simulink model "Copy_of_Robot_PID_Trajectory_Control"  (R2019b)
settings: Solver=VariableStepAuto  StartTime=0.0  StopTime=6  RelTol=1e-3  EnableMultiTasking=on
model workspace: external: MATLAB File D:\Google Drive\Duongw_Folder\Thesis Master\_Model\Delta_Model_ADEPT\SIMCAPE_MULTI_BODY\ADEPT_DELTA_3AXES1\Assem1_ADEPT_HORNET_DataFile.m (data not in the file)
values from neighbouring files (symbols this model uses):
  G = -5    [Assem1_ADEPT_HORNET_DataFile.m]    (also in data_specMotor.m)
  Kb = 0.4    [Assem1_ADEPT_HORNET_DataFile.m]    (also in data_specMotor.m)
  Kd = 15    [Assem1_ADEPT_HORNET_DataFile.m]    (also in data_specMotor.m)
  Ki = 200    [Assem1_ADEPT_HORNET_DataFile.m]    (also in data_specMotor.m)
  Km = 0.7    [Assem1_ADEPT_HORNET_DataFile.m]    (also in data_specMotor.m)
  Kp = 300    [Assem1_ADEPT_HORNET_DataFile.m]    (also in data_specMotor.m)
  La = 0.0062000000000000006    (= 0.0062)    [Assem1_ADEPT_HORNET_DataFile.m]    (also in data_specMotor.m)
  m = zeros(1,3)    [forward.m]    (also in solequa.m = zeros(3,1))
  Ra = 1.8    [Assem1_ADEPT_HORNET_DataFile.m]    (also in data_specMotor.m)
  smiData = struct    [Assem1_ADEPT_HORNET_DataFile.m]
undefined symbols (not defined in the file or in its folder): X, Y, Z
libraries: sm_lib x106, nesl_utility x7
(part 1 of 4)
settings Model: Creator=ThanhUTC  LastModifiedBy=ShiningDanyang
settings DataIOCC: SaveFormat=Array  ReturnWorkspaceOutputs=off
settings OptimizationCC: LifeSpan=inf
settings DebuggingCC: SFUnexpectedBacktrackingDiag=warning  SFNoUnconditionalDefaultTransitionDiag=warning  SFExecutionAtInitializationDiag=none  ArithmeticOperatorsInVariantConditions=warning
settings SFSimCC: SimUseLocalCustomCode=off  CustomCodeUndefinedFunction=UseInterfaceOnly
settings RTWCC: RTWUseLocalCustomCode=off
settings CodeAppCC: StateflowObjectComments=on
settings GRTTargetCC: TargetLangStandard=C89/C90 (ANSI)
settings ConfigComp: CovMetricSettings=dw  CovHtmlReporting=on  CovSaveCumulativeToWorkspaceVar=on  CovSaveSingleToWorkspaceVar=on  CovExternalEMLEnable=off
settings SimscapeCC: SimscapeNormalizeSystem=off
settings ExplorerConfigSet: InternalSimMechanicsExplorerSettings="<ExplorerConfiguration><canonicalview>aerospace</canonicalview><AnimationSetting><BasePlaybackSpeed>1.0</BasePlaybackSpeed><PlaybackSpeedFactor>1.0</PlaybackSpeedFactor></AnimationSetting><TilePanel><TileInfo><Tiles Columns=\"2\" Count=\"4\" Rows=\"2\"><Column Left=\"2\" Weight=\"0.5\"/><Column Left=\"475\" Weight=\"0.5\"/><Column Left=\"948\"/><Row Top=\"2\" Weight=\"0.4991\"/><Row Top=\"300\" Weight=\"0.5009\"/><Row Top=\"599\"/><Tile Height=\"1\" Width=\"1\" X=\"0\" Y=\"0\"/><Tile Height=\"1\" Width=\"1\" X=\"0\" Y=\"1\"/><Tile Height=\"1\" Width=\"1\" X=\"1\" Y=\"0\"/><Tile Height=\"1\" Width=\"1\" X=\"1\" Y=\"1\"/></Tiles></TileInfo><SceneInfo><SceneViewer><BGColor><R>0.60000002384185791</R><G>0.60000002384185791</G><B>0.60000002384185791</B></BGColor><Camera><DoPerspective>off</DoPerspective><Position><X>0.70243808377411976</X><Y>0.13073659989605124</Y><Z>0.39252081211592249</Z></Position><Center><X>-0.2309184998542182</X><Y>0.13073659989605124</Y><Z>0.39252081211592249</Z></Center><Up><X>0</X><Y>0</Y><Z>-1</Z></Up><ViewLimDist>1</ViewLimDist><YLim>0.65085916161537172</YLim><XLim>1.0449780311056487</XLim></Camera></SceneViewer><SceneViewer><BGColor><R>0.60000002384185791</R><G>0.60000002384185791</G><B>0.60000002384185791</B></BGColor><Camera><DoPerspective>off</DoPerspective><Position><X>-0.23091849925817176</X><Y>0.13073659989605124</Y><Z>-0.77434821586150304</Z></Position><Center><X>-0.23091849925817176</X><Y>0.13073659989605124</Y><Z>0.3925208407261519</Z></Center><Up><X>0</X><Y>-1</Y><Z>0</Z></Up><ViewLimDist>1</ViewLimDist><YLim>0.42854619026184082</YLim><XLim>0.68567390441894538</XLim></Camera></SceneViewer><SceneViewer><BGColor><R>0.60000002384185791</R><G>0.60000002384185791</G><B>0.60000002384185791</B></BGColor><Camera><DoPerspective>off</DoPerspective><Position><X>-0.23091849925817176</X><Y>-0.77390347671190962</Y><Z>0.39252081211592216</Z></Position><Center><X>-0.23091849925817176</X><Y>0.13073658559093626</Y><Z>0.39252081211592216</Z></Center><Up><X>0</X><Y>0</Y><Z>-1</Z></Up><ViewLimDist>1</ViewLimDist><YLim>0.65085916161537172</YLim><XLim>1.0449780311056487</XLim></Camera></SceneViewer><SceneViewer><BGColor><R>0.60000002384185791</R><G>0.60000002384185791</G><B>0.60000002384185791</B></BGColor><Camera><DoPerspective>off</DoPerspective><Position><X>0.27338855069047568</X><Y>-0.44960389100580933</Y><Z>-0.34981142573849433</Z></Position><Center><X>-0.23784198094965553</X><Y>0.061626640634321911</Y><Z>0.16141910590163688</Z></Center><Up><X>-0.40824829046386307</X><Y>0.40824829046386307</Y><Z>-0.81649658092772615</Z></Up><ViewLimDist>1</ViewLimDist><YLim>0.7367131638526917</YLim><XLim>1.1787410621643069</XLim></Camera></SceneViewer></SceneInfo></TilePanel><MechEditorPanel><Cameras/><GfxPanelCameraMap/></MechEditorPanel></ExplorerConfiguration>"

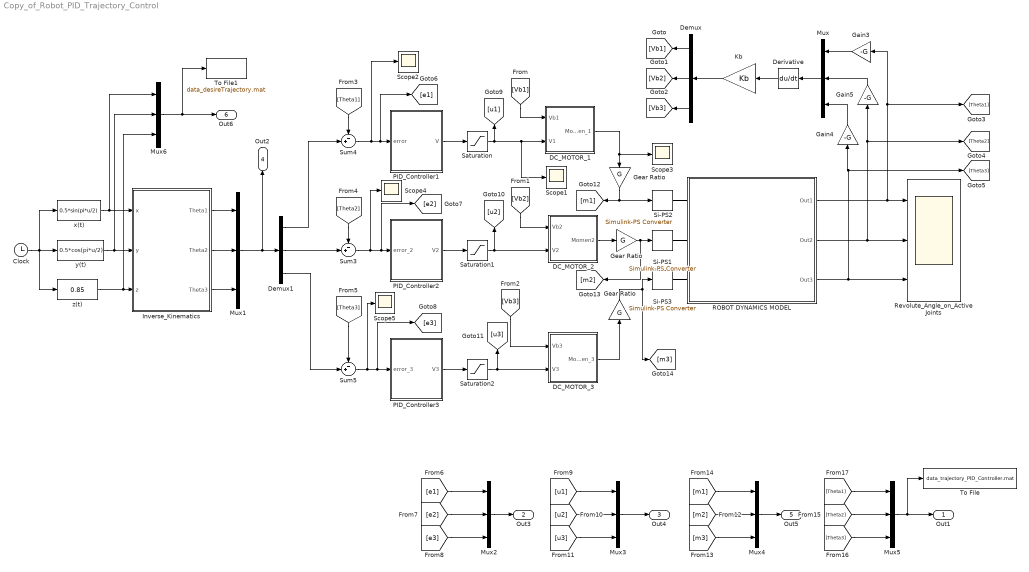
== system Copy_of_Robot_PID_Trajectory_Control ==
  Clock : Clock
  DC_MOTOR_1 : Subsystem
  DC_MOTOR_2 : Subsystem
  DC_MOTOR_3 : Subsystem
  Demux : Demux  Outputs=3
  Demux1 : Demux  Outputs=3
  Derivative : Derivative
  Gain3 : Gain  Gain=-G
  Gain4 : Gain  Gain=-G
  Gain5 : Gain  Gain=-G
  Gear Ratio : Gain  Gain=G
  Gear Ratio : Gain  Gain=G
  "Gear Ratio " : Gain  Gain=G
  Inverse_Kinematics : Subsystem
  Kb : Gain  Gain=Kb
  Mux{,1..6} (7 alike) : Mux  Inputs=3
  PID_Controller1 : Subsystem
  PID_Controller2 : Subsystem
  PID_Controller3 : Subsystem
  ROBOT DYNAMICS MODEL : Subsystem
  Revolute_Angle_on_Active Joints : Scope  NumInputPorts=3
  Saturation : Saturate  UpperLimit=40  LowerLimit=-40  ZeroCross=off
  Saturation1 : Saturate  UpperLimit=40  LowerLimit=-40  ZeroCross=off
  Saturation2 : Saturate  UpperLimit=40  LowerLimit=-40  ZeroCross=off
  Scope{1..5} (5 alike) : Scope
  Si-PS1 : nesl_utility/Simulink-PS Converter  PhysicalDomain=network_engine_domain  SubClassName=ps_input  LeftPortType=input  RightPortType=output  PseudoPeriodic=off  Frequencies=[]  NoiseDistribution=none  NoiseParameters=[]  Unit=1  AffineConversion=off  FilteringAndDerivatives=filter  SimscapeFilterOrder=2  InputFilterTimeConstant=0.001  UdotUserProvided=1
  Si-PS2 : nesl_utility/Simulink-PS Converter  PhysicalDomain=network_engine_domain  SubClassName=ps_input  LeftPortType=input  RightPortType=output  PseudoPeriodic=off  Frequencies=[]  NoiseDistribution=none  NoiseParameters=[]  Unit=1  AffineConversion=off  FilteringAndDerivatives=filter  SimscapeFilterOrder=2  InputFilterTimeConstant=0.001  UdotUserProvided=1
  Si-PS3 : nesl_utility/Simulink-PS Converter  PhysicalDomain=network_engine_domain  SubClassName=ps_input  LeftPortType=input  RightPortType=output  PseudoPeriodic=off  Frequencies=[]  NoiseDistribution=none  NoiseParameters=[]  Unit=1  AffineConversion=off  FilteringAndDerivatives=filter  SimscapeFilterOrder=2  InputFilterTimeConstant=0.001  UdotUserProvided=1
  Sum3 : Sum  Inputs=-+|
  Sum4 : Sum  Inputs=-+|
  Sum5 : Sum  Inputs=-+|
  To File : ToFile  Filename=data_trajectory_PID_Controller.mat
  To File1 : ToFile  Filename=data_desireTrajectory.mat  MatrixName=xyz_d
  x(t) : Fcn  Expr=0.5*sin(pi*u/2)
  y(t) : Fcn  Expr=0.5*cos(pi*u/2)
  z(t) : Fcn  Expr=0.85
  Out1 : Outport  VectorParamsAs1DForOutWhenUnconnected=off
  Out3 : Outport  Port=2  VectorParamsAs1DForOutWhenUnconnected=off
  Out4 : Outport  Port=3  VectorParamsAs1DForOutWhenUnconnected=off
  Out2 : Outport  Port=4  VectorParamsAs1DForOutWhenUnconnected=off
  Out5 : Outport  Port=5  VectorParamsAs1DForOutWhenUnconnected=off
  Out6 : Outport  Port=6  VectorParamsAs1DForOutWhenUnconnected=off
  wires:
  Mux/1 -> Derivative/1
  Derivative/1 -> Kb/1
  Kb/1 -> Demux/1
  Demux/1 -> [Vb1]
  Demux/2 -> [Vb2]
  Demux/3 -> [Vb3]
  [Theta1] -> Sum4/1
  [Vb1] -> DC_MOTOR_1/1(Vb1)
  PID_Controller1/1("V ") -> Saturation/1
  DC_MOTOR_1/1(Momen_1) -> Scope3/1, Gear Ratio/1
  [Theta2] -> Sum3/1
  Sum3/1 -> Scope4/1, [e2], PID_Controller2/1(error_2)
  PID_Controller2/1("V2 ") -> Saturation1/1
  [Theta3] -> Sum5/1
  Sum5/1 -> Scope5/1, [e3], PID_Controller3/1(error_3)
  PID_Controller3/1("V3 ") -> Saturation2/1
  [Vb2] -> DC_MOTOR_2/1(Vb2)
  DC_MOTOR_2/1(Momen2) -> Gear Ratio/1
  [Vb3] -> DC_MOTOR_3/1(Vb3)
  DC_MOTOR_3/1(Momen_3) -> "Gear Ratio "/1
  "Gear Ratio "/1 -> [m3], Si-PS3/1
  Gear Ratio/1 -> Si-PS1/1, [m2]
  ROBOT DYNAMICS MODEL/1(Out1) -> Gain3/1, [Theta1], Revolute_Angle_on_Active Joints/1
  ROBOT DYNAMICS MODEL/2(Out2) -> Revolute_Angle_on_Active Joints/2, Gain5/1, [Theta2]
  ROBOT DYNAMICS MODEL/3(Out3) -> Revolute_Angle_on_Active Joints/3, Gain4/1, [Theta3]
  Gain3/1 -> Mux/1
  Gain4/1 -> Mux/3
  Gain5/1 -> Mux/2
  Demux1/1 -> Sum4/2
  Demux1/2 -> Sum3/2
  Demux1/3 -> Sum5/2
  Clock/1 -> z(t)/1, x(t)/1, y(t)/1
  Inverse_Kinematics/1(Theta1) -> Mux1/1
  Inverse_Kinematics/2(Theta2) -> Mux1/2
  Inverse_Kinematics/3(Theta3) -> Mux1/3
  Mux1/1 -> Out2/1, Demux1/1
  Mux5/1 -> To File/1, Out1/1
  [Theta1] -> Mux5/1
  [Theta2] -> Mux5/2
  [Theta3] -> Mux5/3
  Mux6/1 -> To File1/1, Out6/1
  z(t)/1 -> Mux6/3, Inverse_Kinematics/3(z)
  y(t)/1 -> Mux6/2, Inverse_Kinematics/2(y)
  x(t)/1 -> Mux6/1, Inverse_Kinematics/1(x)
  [e1] -> Mux2/1
  Mux2/1 -> Out3/1
  [e2] -> Mux2/2
  [e3] -> Mux2/3
  Mux3/1 -> Out4/1
  [u2] -> Mux3/2
  [u3] -> Mux3/3
  [u1] -> Mux3/1
  [m3] -> Mux4/3
  Mux4/1 -> Out5/1
  [m2] -> Mux4/2
  [m1] -> Mux4/1
  Sum4/1 -> Scope2/1, [e1], PID_Controller1/1(error)
  Saturation/1 -> [u1], Scope1/1, DC_MOTOR_1/2(V1)
  Saturation1/1 -> [u2], DC_MOTOR_2/2(V2)
  Saturation2/1 -> [u3], DC_MOTOR_3/2(V3)
  Gear Ratio/1 -> Si-PS2/1, [m1]
  connections:
  Si-PS2/RConn1 -- ROBOT DYNAMICS MODEL/LConn1
  Si-PS1/RConn1 -- ROBOT DYNAMICS MODEL/LConn2
  Si-PS3/RConn1 -- ROBOT DYNAMICS MODEL/LConn3

== system Copy_of_Robot_PID_Trajectory_Control/DC_MOTOR_1 ==
  Vb1 : Inport
  V1 : Inport  Port=2
  Gain1 : Gain  Gain=Km
  Sum : Sum  Inputs=-+|
  Transfer Fcn : TransferFcn  Denominator=[La Ra]
  Momen_1 : Outport  VectorParamsAs1DForOutWhenUnconnected=off
  wires:
  Sum/1 -> Transfer Fcn/1
  Transfer Fcn/1 -> Gain1/1
  Gain1/1 -> Momen_1/1
  Vb1/1 -> Sum/1
  V1/1 -> Sum/2

== system Copy_of_Robot_PID_Trajectory_Control/DC_MOTOR_2 ==
  Vb2 : Inport
  V2 : Inport  Port=2
  Gain2 : Gain  Gain=Km
  Sum1 : Sum  Inputs=-+|
  Transfer Fcn1 : TransferFcn  Denominator=[La Ra]
  Momen2 : Outport  VectorParamsAs1DForOutWhenUnconnected=off
  wires:
  Vb2/1 -> Sum1/1
  Transfer Fcn1/1 -> Gain2/1
  Sum1/1 -> Transfer Fcn1/1
  Gain2/1 -> Momen2/1
  V2/1 -> Sum1/2

== system Copy_of_Robot_PID_Trajectory_Control/DC_MOTOR_3 ==
  Vb3 : Inport
  V3 : Inport  Port=2
  Gain3 : Gain  Gain=Km
  Sum2 : Sum  Inputs=-+|
  Transfer Fcn2 : TransferFcn  Denominator=[La Ra]
  Momen_3 : Outport  VectorParamsAs1DForOutWhenUnconnected=off
  wires:
  Vb3/1 -> Sum2/1
  Transfer Fcn2/1 -> Gain3/1
  Sum2/1 -> Transfer Fcn2/1
  Gain3/1 -> Momen_3/1
  V3/1 -> Sum2/2

== system Copy_of_Robot_PID_Trajectory_Control/Inverse_Kinematics ==
  x : Inport
  y : Inport  Port=2
  z : Inport  Port=3
  MATLAB Function : MATLAB Function  TreatAsAtomicUnit=on
  Theta1 : Outport  VectorParamsAs1DForOutWhenUnconnected=off
  Theta2 : Outport  Port=2  VectorParamsAs1DForOutWhenUnconnected=off
  Theta3 : Outport  Port=3  VectorParamsAs1DForOutWhenUnconnected=off
  wires:
  MATLAB Function/3(theta3) -> Theta3/1
  MATLAB Function/2(theta2) -> Theta2/1
  x/1 -> MATLAB Function/1(x)
  y/1 -> MATLAB Function/2(y)
  z/1 -> MATLAB Function/3(z)
  MATLAB Function/1(theta1) -> Theta1/1

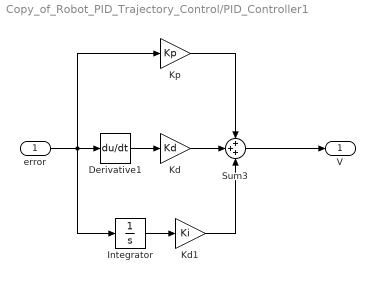
== system Copy_of_Robot_PID_Trajectory_Control/PID_Controller1 ==
  error : Inport
  Derivative1 : Derivative
  Integrator : Integrator
  Kd : Gain  Gain=Kd
  Kd1 : Gain  Gain=Ki
  Kp : Gain  Gain=Kp
  Sum3 : Sum  Inputs=+++
  "V " : Outport  VectorParamsAs1DForOutWhenUnconnected=off
  wires:
  Kd/1 -> Sum3/2
  Kp/1 -> Sum3/1
  Sum3/1 -> "V "/1
  Derivative1/1 -> Kd/1
  error/1 -> Integrator/1, Derivative1/1, Kp/1
  Integrator/1 -> Kd1/1
  Kd1/1 -> Sum3/3

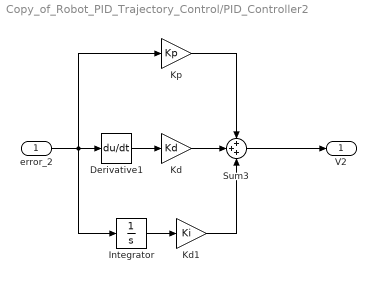
== system Copy_of_Robot_PID_Trajectory_Control/PID_Controller2 ==
  error_2 : Inport
  Derivative1 : Derivative
  Integrator : Integrator
  Kd : Gain  Gain=Kd
  Kd1 : Gain  Gain=Ki
  Kp : Gain  Gain=Kp
  Sum3 : Sum  Inputs=+++
  "V2 " : Outport  VectorParamsAs1DForOutWhenUnconnected=off
  wires:
  Kd1/1 -> Sum3/3
  Integrator/1 -> Kd1/1
  error_2/1 -> Kp/1, Derivative1/1, Integrator/1
  Derivative1/1 -> Kd/1
  Sum3/1 -> "V2 "/1
  Kp/1 -> Sum3/1
  Kd/1 -> Sum3/2

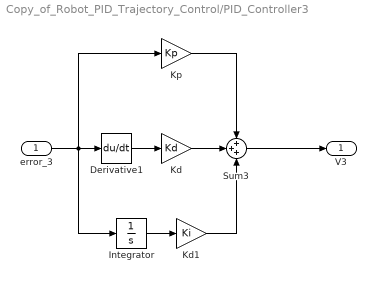
== system Copy_of_Robot_PID_Trajectory_Control/PID_Controller3 ==
  error_3 : Inport
  Derivative1 : Derivative
  Integrator : Integrator
  Kd : Gain  Gain=Kd
  Kd1 : Gain  Gain=Ki
  Kp : Gain  Gain=Kp
  Sum3 : Sum  Inputs=+++
  "V3 " : Outport  VectorParamsAs1DForOutWhenUnconnected=off
  wires:
  Kd/1 -> Sum3/2
  Kp/1 -> Sum3/1
  Sum3/1 -> "V3 "/1
  Derivative1/1 -> Kd/1
  error_3/1 -> Integrator/1, Derivative1/1, Kp/1
  Integrator/1 -> Kd1/1
  Kd1/1 -> Sum3/3
